simulink model "PlantSimulation"  (R2022b)
settings: Solver=FixedStepAuto  StartTime=0.0  StopTime=10  FixedStep=1e-5  RelTol=1e-3
model workspace (MAT data in the model file):
  B_f = Simulink.Parameter
  B_f.Value = 0.0036
  B_f.DataType = 'auto'
  B_f.DocUnits = 'N*m*s'
  B_f.Complexity = 'real'
  B_f.Dimensions = [1 1]
  B_w = Simulink.Parameter
  B_w.Value = 1.93e-05
  B_w.DataType = 'auto'
  B_w.DocUnits = 'kg*m^2'
  B_w.Complexity = 'real'
  B_w.Dimensions = [1 1]
  J_f = Simulink.Parameter
  J_f.Value = 0.0067
  J_f.DataType = 'auto'
  J_f.DocUnits = 'kg*m^2'
  J_f.Complexity = 'real'
  J_f.Dimensions = [1 1]
  J_w = Simulink.Parameter
  J_w.Value = 0.00699
  J_w.DataType = 'auto'
  J_w.DocUnits = 'n*m*s'
  J_w.Complexity = 'real'
  J_w.Dimensions = [1 1]
  g = Simulink.Parameter
  g.Value = 9.816
  g.DataType = 'auto'
  g.DocUnits = 'm/s^2'
  g.Complexity = 'real'
  g.Dimensions = [1 1]
  l_f = Simulink.Parameter
  l_f.Value = 0.0958
  l_f.DataType = 'auto'
  l_f.DocUnits = 'm'
  l_f.Complexity = 'real'
  l_f.Dimensions = [1 1]
  l_w = Simulink.Parameter
  l_w.Value = 0.092
  l_w.DataType = 'auto'
  l_w.DocUnits = 'm'
  l_w.Complexity = 'real'
  l_w.Dimensions = [1 1]
  m_f = Simulink.Parameter
  m_f.Value = 0.819
  m_f.DataType = 'auto'
  m_f.DocUnits = 'kg'
  m_f.Complexity = 'real'
  m_f.Dimensions = [1 1]
  m_w = Simulink.Parameter
  m_w.Value = 0.22
  m_w.DataType = 'auto'
  m_w.DocUnits = 'kg'
  m_w.Complexity = 'real'
  m_w.Dimensions = [1 1]
settings Model: Creator=Sylve  LastModifiedBy=david
settings SolverCC: AlgebraicLoopSolver=TrustRegion
settings DebuggingCC: UnconnectedInputMsg=warning  UnconnectedOutputMsg=warning  UnconnectedLineMsg=warning  SFMachineParentedDataDiag=warning
settings ModelReferenceCC: EnableRefExpFcnMdlSchedulingChecks=on

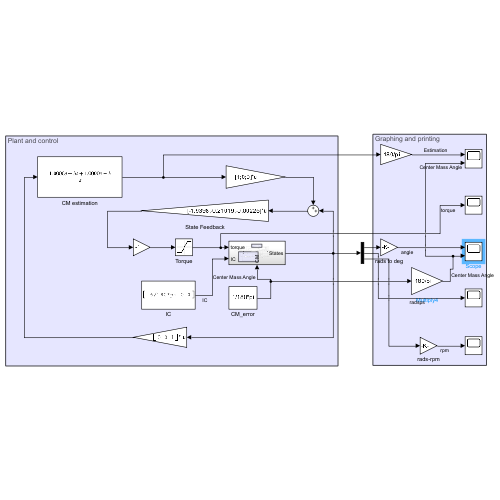
[thumbnail: Simulink's stored preview of the top-level diagram]
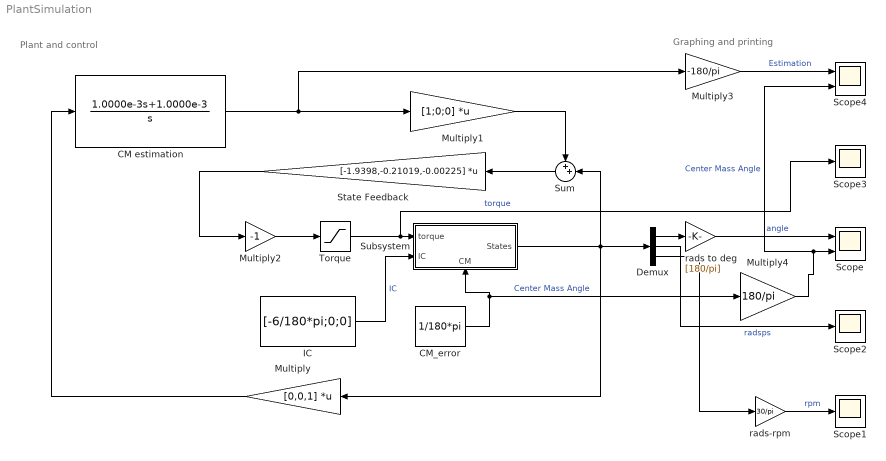
== system PlantSimulation ==
  note: Graphing and printing
  note: Plant and control
  CM estimation : TransferFcn  Numerator=[1.0000e-3 1.0000e-3]  Denominator=[1 0]
  CM_error : Constant  Value=1/180*pi
  Demux : Demux  Outputs=3
  IC : Constant  Value=[-6/180*pi;0;0]
  Multiply : Gain  Gain=[0,0,1]  Multiplication=Matrix(K*u)
  Multiply1 : Gain  Gain=[1;0;0]  Multiplication=Matrix(K*u)
  Multiply2 : Gain  Gain=-1
  Multiply3 : Gain  Gain=-180/pi
  Multiply4 : Gain  Gain=180/pi
  Scope : Scope  NumInputPorts=2
  Scope1 : Scope
  Scope2 : Scope
  Scope3 : Scope
  Scope4 : Scope  NumInputPorts=2
  State Feedback : Gain  Gain=[-1.9398,-0.21019,-0.00225]  Multiplication=Matrix(K*u)
  Subsystem : Subsystem
      settings: PortSchema="{\"entries\":[{\"content\":{\"sides\":[{\"content\":{\"connectorIds\":[\"In1\",\"In2\"]},\"type\":\"ConnectorPlacement.EquallySpacedRectSide\",\"uuid\":\"e7061c55-2b62-4262-b0e7-7a5bab08f6b1\"},{\"content\":{\"connectorIds\":[\"Out1\"],\"side\":\"RIGHT\"},\"type\":\"ConnectorPlacement.EquallySpacedRectSide\",\"uuid\":\"5d6af3c2-eba8-48f3-a8f1-c49dd0c9c08f\"},{\"content\":{\"connectorIds\":[],\"side\":\"TOP\"},\"type\":\"ConnectorPlacement.EquallySpacedRectSide\",\"uuid\":\"5b12f7b1-8495-4110-99ef-78eef5a35a26\"},{\"content\":{\"connectorIds\":[\"In3\"],\"side\":\"BOTTOM\"},\"type\":\"ConnectorPlacement.EquallySpacedRectSide\",\"uuid\":\"c0be89a2-79ad-4613-a652-71050285bf40\"}]},\"type\":\"ConnectorPlacement.EquallySpacedConnector\",\"uuid\":\"06b6dccf-8436-4f6a-8177-d27750d6e3eb\"}],\"packageUris\":[\"http://schema.mathworks.com/mf0/Connector/R2020b\"],\"version\":\"1.0\"}"
  Sum : Sum  Inputs=++|
  Torque : Saturate  UpperLimit=4*33.5/1000  LowerLimit=-4*33.5/1000
  rads to deg : Gain  Gain=[180/pi]
  rads-rpm : Gain  Gain=30/pi
  wires:
  IC/1 -> Subsystem/2(IC)  "IC"
  Subsystem/1(States) -> Multiply/1, Demux/1, Sum/2
  State Feedback/1 -> Multiply2/1
  rads to deg/1 -> Scope/1  "angle"
  Demux/1 -> rads to deg/1
  Demux/3 -> rads-rpm/1
  rads-rpm/1 -> Scope1/1  "rpm"
  Demux/2 -> Scope2/1  "radsps"
  Torque/1 -> Scope3/1, Subsystem/1(torque)  "torque"
  CM estimation/1 -> Multiply3/1, Multiply1/1
  Multiply/1 -> CM estimation/1
  Sum/1 -> State Feedback/1
  Multiply1/1 -> Sum/1
  Multiply2/1 -> Torque/1
  Multiply3/1 -> Scope4/1  "Estimation"
  CM_error/1 -> Subsystem/3(CM), Multiply4/1  "Center Mass Angle"
  Multiply4/1 -> Scope4/2, Scope/2  "Center Mass Angle"

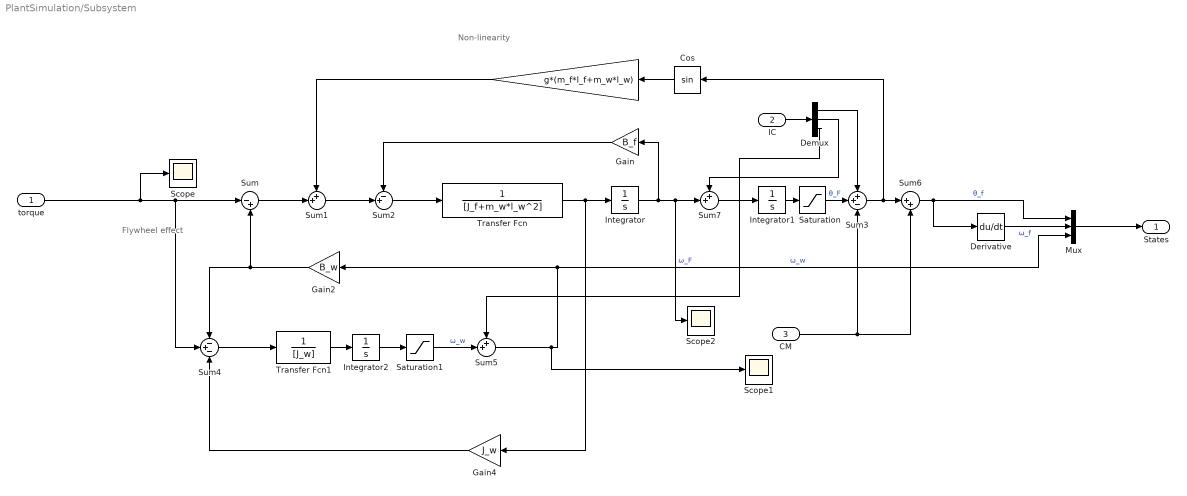
== system PlantSimulation/Subsystem ==
  note: Non-linearity
  note: Flywheel effect
  torque : Inport
  IC : Inport  Port=2
  CM : Inport  Port=3
  " " : Gain  Gain=g*(m_f*l_f+m_w*l_w)
  Cos : Trigonometry
  Demux : Demux  Outputs=3
  Derivative : Derivative
  Gain : Gain  Gain=B_f
  Gain2 : Gain  Gain=B_w
  Gain4 : Gain  Gain=J_w
  Integrator : Integrator
  Integrator1 : Integrator
  Integrator2 : Integrator
  Mux : Mux  Inputs=3
  Saturation : Saturate  UpperLimit=45/180*pi  LowerLimit=-45/180*pi
  Saturation1 : Saturate  UpperLimit=6000  LowerLimit=-6000
  Scope : Scope
  Scope1 : Scope
  Scope2 : Scope
  Sum : Sum  Inputs=|-+
  Sum1 : Sum  Inputs=++|
  Sum2 : Sum  Inputs=-+|
  Sum3 : Sum  Inputs=++-
  Sum4 : Sum  Inputs=-+-
  Sum5 : Sum  Inputs=++|
  Sum6 : Sum  Inputs=|++
  Sum7 : Sum  Inputs=++|
  Transfer Fcn : TransferFcn  Denominator=[J_f+m_w*l_w^2]
  Transfer Fcn1 : TransferFcn  Denominator=[J_w]
  States : Outport  PortDimensions=3
  wires:
  Transfer Fcn/1 -> Gain4/1, Integrator/1
  Integrator2/1 -> Saturation1/1
  Gain4/1 -> Sum4/3
  Gain/1 -> Sum2/1
  Transfer Fcn1/1 -> Integrator2/1
  Sum4/1 -> Transfer Fcn1/1
  Sum5/1 -> Scope1/1, Mux/3, Gain2/1  "ω_w"
  Integrator/1 -> Scope2/1, Sum7/2, Gain/1  "ω_F"
  Sum1/1 -> Sum2/2
  Sum2/1 -> Transfer Fcn/1
  " "/1 -> Sum1/1
  Sum/1 -> Sum1/2
  Integrator1/1 -> Saturation/1
  IC/1 -> Demux/1
  Sum3/1 -> Sum6/1, Cos/1
  Mux/1 -> States/1
  Sum6/1 -> Derivative/1, Mux/1  "θ_f"
  CM/1 -> Sum6/2, Sum3/3
  Saturation/1 -> Sum3/2  "θ_F"
  Derivative/1 -> Mux/2  "ω_f"
  Cos/1 -> " "/1
  torque/1 -> Scope/1, Sum/1, Sum4/2
  Demux/1 -> Sum3/1
  Sum7/1 -> Integrator1/1
  Demux/2 -> Sum7/1
  Gain2/1 -> Sum4/1, Sum/2
  Saturation1/1 -> Sum5/2  "ω_w"
  Demux/3 -> Sum5/1
